simulink model "dynamic1"  (R2019a)
settings: Solver=VariableStepAuto  StartTime=0.0  StopTime=10.0  RelTol=1e-3
libraries: simulink x2
settings Model: Creator=ChairmanYang1966  LastModifiedBy=ChairmanYang1966

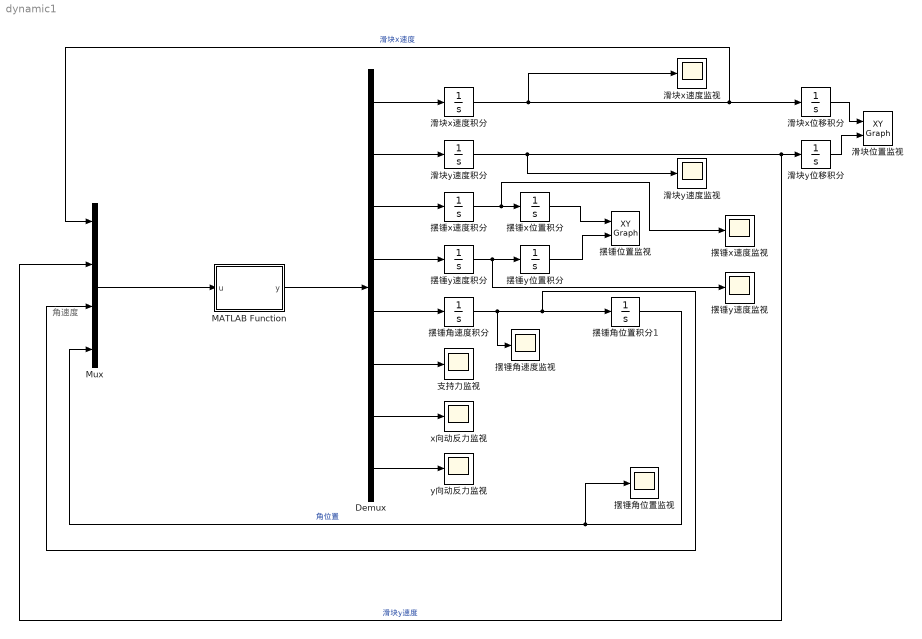
== system dynamic1 ==
  note: 角速度
  Demux : Demux  Outputs=8
  MATLAB Function : MATLAB Function  TreatAsAtomicUnit=on
  Mux : Mux
  x向动反力监视 : Scope
  y向动反力监视 : Scope
  摆锤x位置积分 : Integrator  InitialCondition=0.3536
  摆锤x速度监视 : Scope
  摆锤x速度积分 : Integrator
  摆锤y位置积分 : Integrator  InitialCondition=0.6464
  摆锤y速度监视 : Scope
  摆锤y速度积分 : Integrator
  摆锤位置监视 : simulink/Sinks/XY Graph  xmin=-2  xmax=2  ymin=-2  ymax=2  st=-1
  摆锤角位置监视 : Scope
  摆锤角位置积分1 : Integrator  InitialCondition=-pi/4
  摆锤角速度监视 : Scope
  摆锤角速度积分 : Integrator
  支持力监视 : Scope
  滑块x位移积分 : Integrator
  滑块x速度监视 : Scope
  滑块x速度积分 : Integrator
  滑块y位移积分 : Integrator  InitialCondition=1
  滑块y速度监视 : Scope
  滑块y速度积分 : Integrator
  滑块位置监视 : simulink/Sinks/XY Graph  xmin=-2  xmax=2  ymin=-2  ymax=2  st=-1
  wires:
  Mux/1 -> MATLAB Function/1(u)
  MATLAB Function/1(y) -> Demux/1
  Demux/1 -> 滑块x速度积分/1
  Demux/2 -> 滑块y速度积分/1
  滑块y速度积分/1 -> 滑块y速度监视/1, Mux/2, 滑块y位移积分/1  "滑块y速度"
  滑块x速度积分/1 -> 滑块x速度监视/1, Mux/1, 滑块x位移积分/1  "滑块x速度"
  滑块x位移积分/1 -> 滑块位置监视/1
  Demux/4 -> 摆锤y速度积分/1
  Demux/3 -> 摆锤x速度积分/1
  摆锤x速度积分/1 -> 摆锤x速度监视/1, 摆锤x位置积分/1
  摆锤y速度积分/1 -> 摆锤y速度监视/1, 摆锤y位置积分/1
  Demux/5 -> 摆锤角速度积分/1
  Demux/6 -> 支持力监视/1
  Demux/7 -> x向动反力监视/1
  Demux/8 -> y向动反力监视/1
  摆锤x位置积分/1 -> 摆锤位置监视/1
  摆锤y位置积分/1 -> 摆锤位置监视/2
  摆锤角速度积分/1 -> 摆锤角位置积分1/1, Mux/3, 摆锤角速度监视/1
  摆锤角位置积分1/1 -> 摆锤角位置监视/1, Mux/4  "角位置"
  滑块y位移积分/1 -> 滑块位置监视/2

== matlab function dynamic1/MATLAB Function ==
  data: u input; y output
function y = fcn(u)
m1=5;m2=0.5;J=0.01;a=pi/6;l=0.5;g=9.8687;mu=0.5;
v=u(1)*cos(a)-u(2)*sin(a);
if v>0
    sigma=1.0;
else
    sigma=-1.0;
end
b=[0;-m1*g;0;-m2*g;0;l*u(3)^2*cos(u(4));l*u(3)^2*sin(u(4));0];
A=[m1 0 0 0 0 sigma*mu*cos(a)-sin(a) 1 0;
    0 m1 0 0 0 -sigma*mu*sin(a)-cos(a) 0 1;
    0 0 m2 0 0 0 -1 0;
    0 0 0 m2 0 0 0 -1
    0 0 0 0 J 0 -l*sin(u(4)) l*cos(u(4));
    1 0 -1 0 -l*sin(u(4)) 0 0 0;
    0 1 0 -1 l*cos(u(4)) 0 0 0;
    sin(a) cos(a) 0 0 0 0 0 0];
y = inv(A)*b;
%滑块质量5kg，摆锤质量5kg，摩擦因数0.5，重力加速度取9.8687m/s2；斜面倾角30度
%摆锤转动惯量0.01kgm2，摆锤长0.5m，滑块初始高度1m，x坐标为0，摆锤初始摆角45度
%u(1),u(2)分别是滑块的x,y向速度，u(3)为摆锤角速度，u(4)为摆锤角位置
%y(1),y(2)分别是滑块的x,y向加速度，y(3),y(4)分别是摆锤的x,y向加速度
%y(5)为摆锤的角加速度，y(6),y(7),y(8)分别是滑块支持力，滑块-摆锤系统内部的x,y向动反力
